simulink model "v2x_cs"  (R2019a)
settings: Solver=ode5  StartTime=0.0  StopTime=inf  FixedStep=1/20  RelTol=1e-3
PreLoadFcn:
  | mbxruntime.callbacks.PreLoadFcn(bdroot);
PostLoadFcn:
  | mbxruntime.callbacks.PostLoadFcn(bdroot);
InitFcn:
  | mbxruntime.callbacks.InitFcn(bdroot);
StartFcn:
  | mbxruntime.callbacks.StartFcn(bdroot);
StopFcn:
  | mbxruntime.callbacks.StopFcn(bdroot);
model workspace (MAT data in the model file):
  mbox_table : struct (value not decoded)
  model_closed = 0
  sim_status = 0
undefined symbols (not defined in the file or in its folder): DiscIntNeverNeededParam, SteeringWheel
libraries: PreScanSimulinkLibrary x10
(part 1 of 5)
CloseFcn:
  | mbxruntime.callbacks.CloseFcn(bdroot);
settings Model: Creator=PRESCAN  LastModifiedBy=DELL
settings DataIOCC: LimitDataPoints=on  SaveFormat=Array  SignalLoggingSaveFormat=ModelDataLogs  ReturnWorkspaceOutputs=off
settings OptimizationCC: ExpressionDepthLimit=2147483647  InitFltsAndDblsToZero=on  LifeSpan=inf
settings DebuggingCC: SaveWithParameterizedLinksMsg=none  UnderspecifiedInitializationDetection=Classic  MergeDetectMultiDrivingBlocksExec=none  SignalResolutionControl=TryResolveAllWithWarning  MultiTaskDSMMsg=warning  MultiTaskCondExecSysMsg=none  FcnCallInpInsideContextMsg=warning  StateNameClashWarn=warning  SFUnexpectedBacktrackingDiag=warning  SFNoUnconditionalDefaultTransitionDiag=warning  SFExecutionAtInitializationDiag=none  ArithmeticOperatorsInVariantConditions=warning
settings HardwareCC: ProdBitPerPointer=32  ProdBitPerSizeT=32  ProdBitPerPtrDiffT=32  ProdLargestAtomicFloat=None  ProdIntDivRoundTo=Undefined  ProdEndianess=Unspecified  ProdWordSize=32  ProdHWDeviceType=32-bit Generic
settings ModelReferenceCC: UpdateModelReferenceTargets=IfOutOfDate  PropagateSignalLabelsOutOfModel=off
settings SFSimCC: SimUseLocalCustomCode=off  SimParseCustomCode=off
settings SFSimCC: SimCustomHeaderCode=|
  | #include "prescan.h"
  | #include "prescan_platform.h"
  | #include "prescan_v2x_data.h"
settings RTWCC: RTWUseLocalCustomCode=off
settings CodeAppCC: StateflowObjectComments=on
settings GRTTargetCC: TargetFcnLib=ansi_tfl_tmw.mat  TargetLangStandard=C89/C90 (ANSI)  GeneratePreprocessorConditionals=Disable all  CombineOutputUpdateFcns=off  GRTInterface=on
settings ConfigComp: CovMetricSettings=dw  CovHtmlReporting=on  CovSaveCumulativeToWorkspaceVar=on  CovSaveSingleToWorkspaceVar=on  CovExternalEMLEnable=off

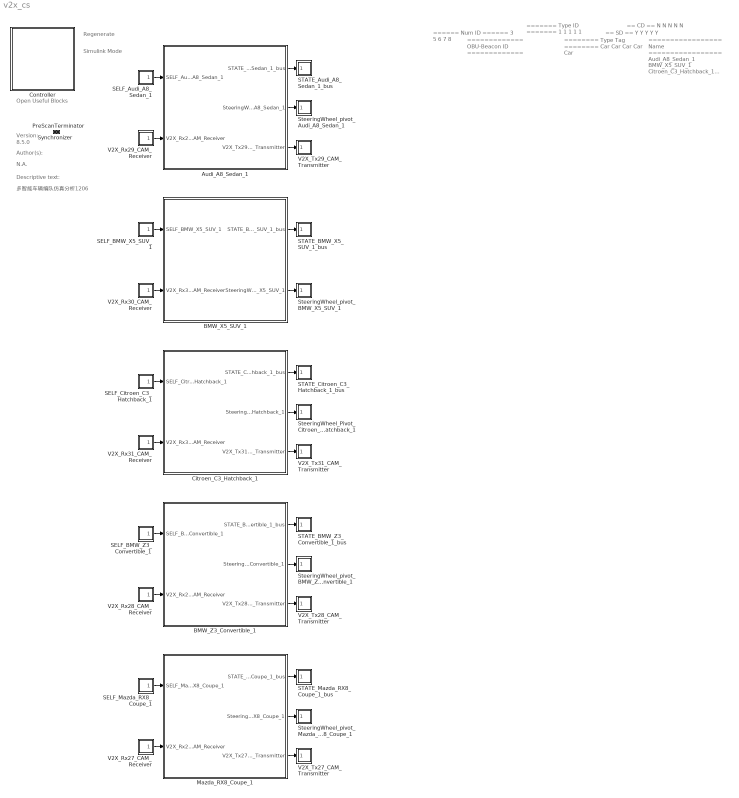
== system v2x_cs ==
  note: Regenerate
  note: Simulink Mode
  note: Open Useful Blocks
  note: 8.5.0
  note: Version:
  note: Author(s):
  note: N.A.
  note: Descriptive text:
  note: 多智能车辆编队仿真分析1206
  note: ======
      | Num ID
      | ======
      | 3
      | 5
      | 6
      | 7
      | 8
  note: =============
      | OBU-Beacon ID
      | =============
  note: =======
      | Type ID
      | =======
      | 1
      | 1
      | 1
      | 1
      | 1
  note: ========
      | Type Tag
      | ========
      | Car
      | Car
      | Car
      | Car
      | Car
  note: ==
      | SD
      | ==
      | Y
      | Y
      | Y
      | Y
      | Y
  note: ==
      | CD
      | ==
      | N
      | N
      | N
      | N
      | N
  note: =================
      | Name
      | =================
      | Audi_A8_Sedan_1
      | BMW_X5_SUV_1
      | Citroen_C3_Hatchback_1
      | BMW_Z3_Convertible_1
      | Mazda_RX8_Coupe_1
  Audi_A8_Sedan_1 : Subsystem  Tag=WorldObjectSubSystem  InitFcn=UniqueId = '22';
      mask init:
      | modelPath = GenericModelHelper.getGenericModelFilePath('ModelDepo','Vehicles\Audi_A8\Audi_A8.pgmb','d771622804618130053427da08a6d484');imagePath = GenericModelHelper.getCompilationPicture(modelPath, 'Audi_A8_HighPoly.png');
      mask Display: image(imread(imagePath));color('white');text(0, 0, ' ID=3\n')
  BMW_X5_SUV_1 : Subsystem  Tag=WorldObjectSubSystem  InitFcn=UniqueId = '23';
      mask init:
      | modelPath = GenericModelHelper.getGenericModelFilePath('ModelDepo','Vehicles\BMW_X5\BMW_X5.pgmb','cea918691563e9ae3e6a88ec95e6726a');imagePath = GenericModelHelper.getCompilationPicture(modelPath, 'BMW_X5_HighPoly.png');
      mask Display: image(imread(imagePath));color('white');text(0, 0, ' ID=5\n')
  BMW_Z3_Convertible_1 : Subsystem  Tag=WorldObjectSubSystem  InitFcn=UniqueId = '25';
      mask init:
      | modelPath = GenericModelHelper.getGenericModelFilePath('ModelDepo','Vehicles\BMW_Z3\BMW_Z3.pgmb','7699e47834166b94c09717861bab4f7a');imagePath = GenericModelHelper.getCompilationPicture(modelPath, 'BMW_Z3_HighPoly.png');
      mask Display: image(imread(imagePath));color('white');text(0, 0, ' ID=7\n')
  Citroen_C3_Hatchback_1 : Subsystem  Tag=WorldObjectSubSystem  InitFcn=UniqueId = '24';
      mask init:
      | modelPath = GenericModelHelper.getGenericModelFilePath('ModelDepo','Vehicles\Citroen_C3\Citroen_C3.pgmb','418afd416d9cb26f62eb87df85de2ab6');imagePath = GenericModelHelper.getCompilationPicture(modelPath, 'Citroen_C3_HighPoly.png');
      mask Display: image(imread(imagePath));color('white');text(0, 0, ' ID=6\n')
  Controller : Subsystem  Description=4395E09780732EACEA18EB3ED2FF7C1B9BEC15E9AB79396025191FD1491BD270  Priority=-1  LoadFcn=load PreScanControllerData  mask(PreScan Simulation Controller){prescanversion='8.5.0', ModelReferencing=off, TimeStep=1/20, ControlMode=0, PreScanExecutionMode=on, ControllerCount=0, ControllerIndex=0, ControllerOptions=''}
      mask prompts: prescanversion "PreScan Version"; ModelReferencing "Use Model Referencing"; TimeStep "Upload Period [s]"; ControlMode "Control Mode"; PreScanExecutionMode "Execution Mode"; ControllerCount "Controller Count"; ControllerIndex "Controller Index"; ControllerOptions "Controller Options"
      mask help:
      | Please do not remove this block from the compilation sheet,
      | as it connects the model to the PreScan environment.
      mask init:
      | model = bdroot(gcb);
      | ExperimentFile = mbxruntime.findExperimentFile(model,true); %relative path
      | 
      | [d1, d2, d3, prescandata] = prescan_Settings();
      | ModelDepo = fullfile(prescandata,'ModelDepo'); 
      | 
      | RTmode = mbxruntime.getRTMode(model);
      | 
      | SimulationMode = get_param(bdroot,'SimulationMode');
      | if strcmp(SimulationMode, 'rapid-accelerator')
      |     SimulationMode = 'external';
      | end
      | TargetName = get_param(bdroot,'SystemTargetFile');
      settings: ModelCloseFcn=assignin('base',['model_closed_' bdroot],true);
      mask Help: eval('openHelp(812)')
      mask Display: image(imread('prescanlogo.ico'))
  Mazda_RX8_Coupe_1 : Subsystem  Tag=WorldObjectSubSystem  InitFcn=UniqueId = '26';
      mask init:
      | modelPath = GenericModelHelper.getGenericModelFilePath('ModelDepo','Vehicles\Mazda_RX8\Mazda_RX8.pgmb','f45c3d42338784d01091d029fcd57bfb');imagePath = GenericModelHelper.getCompilationPicture(modelPath, 'Mazda_RX8_HighPoly.png');
      mask Display: image(imread(imagePath));color('white');text(0, 0, ' ID=8\n')
  PreScanTerminator : Subsystem  Tag=PreScanTerminator  Priority=999  LoadFcn=load PrescanTerminatorData  mask(PreScan Simulation Terminator){TimeStep=1/20}
      mask prompts: TimeStep "Upload Period [s]"
      mask help:
      | Please do not remove this block from the compilation sheet as it
      | connects the model to the PreScan environment.
      mask Help: eval('openHelp(812)')
      mask Display: image(imread('prescanlogo.ico'))
  SELF_Audi_A8_Sedan_1 : Subsystem  Tag=sensor/SelfPort  Priority=3  LoadFcn=load('PreScanSelfSensorData.mat')  mask(PreScan Source Block: SELF){}
      mask help:
      | The SELF port shows (state) information of the actor itself. The outputs are position in the experiment's axis system and the GPS coordinates, and the object's absolute velocity and compass heading.
      |
      | For more information, please click Help.
      settings: OpenFcn=open_system([gcb '/Sensor'],'mask')
      mask Help: eval('openHelp(462)')
      mask Display: image(imread('GPS.png'))
  SELF_BMW_X5_SUV_1 : Subsystem  Tag=sensor/SelfPort  Priority=3  LoadFcn=load('PreScanSelfSensorData.mat')  mask(PreScan Source Block: SELF){}
      mask help:
      | The SELF port shows (state) information of the actor itself. The outputs are position in the experiment's axis system and the GPS coordinates, and the object's absolute velocity and compass heading.
      |
      | For more information, please click Help.
      settings: OpenFcn=open_system([gcb '/Sensor'],'mask')
      mask Help: eval('openHelp(462)')
      mask Display: image(imread('GPS.png'))
  SELF_BMW_Z3_Convertible_1 : Subsystem  Tag=sensor/SelfPort  Priority=3  LoadFcn=load('PreScanSelfSensorData.mat')  mask(PreScan Source Block: SELF){}
      mask help:
      | The SELF port shows (state) information of the actor itself. The outputs are position in the experiment's axis system and the GPS coordinates, and the object's absolute velocity and compass heading.
      |
      | For more information, please click Help.
      settings: OpenFcn=open_system([gcb '/Sensor'],'mask')
      mask Help: eval('openHelp(462)')
      mask Display: image(imread('GPS.png'))
  SELF_Citroen_C3_Hatchback_1 : Subsystem  Tag=sensor/SelfPort  Priority=3  LoadFcn=load('PreScanSelfSensorData.mat')  mask(PreScan Source Block: SELF){}
      mask help:
      | The SELF port shows (state) information of the actor itself. The outputs are position in the experiment's axis system and the GPS coordinates, and the object's absolute velocity and compass heading.
      |
      | For more information, please click Help.
      settings: OpenFcn=open_system([gcb '/Sensor'],'mask')
      mask Help: eval('openHelp(462)')
      mask Display: image(imread('GPS.png'))
  SELF_Mazda_RX8_Coupe_1 : Subsystem  Tag=sensor/SelfPort  Priority=3  LoadFcn=load('PreScanSelfSensorData.mat')  mask(PreScan Source Block: SELF){}
      mask help:
      | The SELF port shows (state) information of the actor itself. The outputs are position in the experiment's axis system and the GPS coordinates, and the object's absolute velocity and compass heading.
      |
      | For more information, please click Help.
      settings: OpenFcn=open_system([gcb '/Sensor'],'mask')
      mask Help: eval('openHelp(462)')
      mask Display: image(imread('GPS.png'))
  STATE_Audi_A8_Sedan_1_bus : Subsystem  Tag=actuator/StatePort  Priority=0  LoadFcn=load('PreScanStateActuatorData.mat')  mask(PreScan Sink Block: State){}
      mask help:
      | The Actor State contains a vector signal of size (9x1), containing the following signals:
      |
      | -  Position    	(x,y,z)             	[m]
      | -  Velocity    	(vx,vy,vz)         	[m/s]
      | -  Angles       	(Roll, Pitch, Yaw)	[rad]
      |
      | The Actor state is defined in the global axis system.
      | The state is superponed on the Initial position defined in the GUI.
      |
      | For more information, please click Help.
      settings: OpenFcn=open_system([gcb '/Actuator'],'mask')
      mask Help: eval('openHelp(222)')
      mask Display: image(imread('State.png'))
  STATE_BMW_X5_SUV_1_bus : Subsystem  Tag=actuator/StatePort  Priority=0  LoadFcn=load('PreScanStateActuatorData.mat')  mask(PreScan Sink Block: State){}
      mask help:
      | The Actor State contains a vector signal of size (9x1), containing the following signals:
      |
      | -  Position    	(x,y,z)             	[m]
      | -  Velocity    	(vx,vy,vz)         	[m/s]
      | -  Angles       	(Roll, Pitch, Yaw)	[rad]
      |
      | The Actor state is defined in the global axis system.
      | The state is superponed on the Initial position defined in the GUI.
      |
      | For more information, please click Help.
      settings: OpenFcn=open_system([gcb '/Actuator'],'mask')
      mask Help: eval('openHelp(222)')
      mask Display: image(imread('State.png'))
  STATE_BMW_Z3_Convertible_1_bus : Subsystem  Tag=actuator/StatePort  Priority=0  LoadFcn=load('PreScanStateActuatorData.mat')  mask(PreScan Sink Block: State){}
      mask help:
      | The Actor State contains a vector signal of size (9x1), containing the following signals:
      |
      | -  Position    	(x,y,z)             	[m]
      | -  Velocity    	(vx,vy,vz)         	[m/s]
      | -  Angles       	(Roll, Pitch, Yaw)	[rad]
      |
      | The Actor state is defined in the global axis system.
      | The state is superponed on the Initial position defined in the GUI.
      |
      | For more information, please click Help.
      settings: OpenFcn=open_system([gcb '/Actuator'],'mask')
      mask Help: eval('openHelp(222)')
      mask Display: image(imread('State.png'))
  STATE_Citroen_C3_Hatchback_1_bus : Subsystem  Tag=actuator/StatePort  Priority=0  LoadFcn=load('PreScanStateActuatorData.mat')  mask(PreScan Sink Block: State){}
      mask help:
      | The Actor State contains a vector signal of size (9x1), containing the following signals:
      |
      | -  Position    	(x,y,z)             	[m]
      | -  Velocity    	(vx,vy,vz)         	[m/s]
      | -  Angles       	(Roll, Pitch, Yaw)	[rad]
      |
      | The Actor state is defined in the global axis system.
      | The state is superponed on the Initial position defined in the GUI.
      |
      | For more information, please click Help.
      settings: OpenFcn=open_system([gcb '/Actuator'],'mask')
      mask Help: eval('openHelp(222)')
      mask Display: image(imread('State.png'))
  STATE_Mazda_RX8_Coupe_1_bus : Subsystem  Tag=actuator/StatePort  Priority=0  LoadFcn=load('PreScanStateActuatorData.mat')  mask(PreScan Sink Block: State){}
      mask help:
      | The Actor State contains a vector signal of size (9x1), containing the following signals:
      |
      | -  Position    	(x,y,z)             	[m]
      | -  Velocity    	(vx,vy,vz)         	[m/s]
      | -  Angles       	(Roll, Pitch, Yaw)	[rad]
      |
      | The Actor state is defined in the global axis system.
      | The state is superponed on the Initial position defined in the GUI.
      |
      | For more information, please click Help.
      settings: OpenFcn=open_system([gcb '/Actuator'],'mask')
      mask Help: eval('openHelp(222)')
      mask Display: image(imread('State.png'))
  SteeringWheel_Pivot_Citroen_C3_Hatchback_1 : Subsystem  Tag=Actuator  Priority=0  LoadFcn=load('PrescanPoseData');load('PrescanXYZData');load('PreScanRPYData')
      mask help:
      | The VisuJoint block provides a way to adapt the location and orientation of a part of an object.
      |
      | For more information, please click Help.
      settings: OpenFcn=open_system([gcb '/Actuator'],'mask')
      mask Display: image(imread('Joint.png'))
  SteeringWheel_pivot_Audi_A8_Sedan_1 : Subsystem  Tag=Actuator  Priority=0  LoadFcn=load('PrescanPoseData');load('PrescanXYZData');load('PreScanRPYData')
      mask help:
      | The VisuJoint block provides a way to adapt the location and orientation of a part of an object.
      |
      | For more information, please click Help.
      settings: OpenFcn=open_system([gcb '/Actuator'],'mask')
      mask Display: image(imread('Joint.png'))
  SteeringWheel_pivot_BMW_X5_SUV_1 : Subsystem  Tag=Actuator  Priority=0  LoadFcn=load('PrescanPoseData');load('PrescanXYZData');load('PreScanRPYData')
      mask help:
      | The VisuJoint block provides a way to adapt the location and orientation of a part of an object.
      |
      | For more information, please click Help.
      settings: OpenFcn=open_system([gcb '/Actuator'],'mask')
      mask Display: image(imread('Joint.png'))
  SteeringWheel_pivot_BMW_Z3_Convertible_1 : Subsystem  Tag=Actuator  Priority=0  LoadFcn=load('PrescanPoseData');load('PrescanXYZData');load('PreScanRPYData')
      mask help:
      | The VisuJoint block provides a way to adapt the location and orientation of a part of an object.
      |
      | For more information, please click Help.
      settings: OpenFcn=open_system([gcb '/Actuator'],'mask')
      mask Display: image(imread('Joint.png'))
  SteeringWheel_pivot_Mazda_RX8_Coupe_1 : Subsystem  Tag=Actuator  Priority=0  LoadFcn=load('PrescanPoseData');load('PrescanXYZData');load('PreScanRPYData')
      mask help:
      | The VisuJoint block provides a way to adapt the location and orientation of a part of an object.
      |
      | For more information, please click Help.
      settings: OpenFcn=open_system([gcb '/Actuator'],'mask')
      mask Display: image(imread('Joint.png'))
  Synchronizer : Subsystem  Tag=PreScanSynchronizer  Priority=1  LoadFcn=load PrescanSynchronizeData  mask(PreScan Simulation Core Block){TimeStep=1/20}
      mask prompts: TimeStep "Timestep [s]"
      mask help:
      | Please do not remove this block from the PreScan compilation sheet,
      | as it contains essential configuration parameters for a PreScan simulation.
      settings: DeleteFcn=PreScanBlockDeleteFcn;
      mask Display: image(imread('prescanlogo.ico'))
  V2X_Rx27_CAM_Receiver : Subsystem  Tag=sensor/plugin/sfun_V2X_CAM_Receiver  Priority=3  mask(V2X CAM Receiver Block){}
      mask help: V2X Block receiving a CAM message
      settings: OpenFcn=open_system([gcb '/Sensor'],'mask')
      mask Help: eval('openHelp()')
      mask Display: image(imread('V2XR_grayscale.png'))
  V2X_Rx28_CAM_Receiver : Subsystem  Tag=sensor/plugin/sfun_V2X_CAM_Receiver  Priority=3  mask(V2X CAM Receiver Block){}
      mask help: V2X Block receiving a CAM message
      settings: OpenFcn=open_system([gcb '/Sensor'],'mask')
      mask Help: eval('openHelp()')
      mask Display: image(imread('V2XR_grayscale.png'))
  V2X_Rx29_CAM_Receiver : Subsystem  Tag=sensor/plugin/sfun_V2X_CAM_Receiver  Priority=3  mask(V2X CAM Receiver Block){}
      mask help: V2X Block receiving a CAM message
      settings: OpenFcn=open_system([gcb '/Sensor'],'mask')
      mask Help: eval('openHelp()')
      mask Display: image(imread('V2XR_grayscale.png'))
  V2X_Rx30_CAM_Receiver : Subsystem  Tag=sensor/plugin/sfun_V2X_CAM_Receiver  Priority=3  mask(V2X CAM Receiver Block){}
      mask help: V2X Block receiving a CAM message
      settings: OpenFcn=open_system([gcb '/Sensor'],'mask')
      mask Help: eval('openHelp()')
      mask Display: image(imread('V2XR_grayscale.png'))
  V2X_Rx31_CAM_Receiver : Subsystem  Tag=sensor/plugin/sfun_V2X_CAM_Receiver  Priority=3  mask(V2X CAM Receiver Block){}
      mask help: V2X Block receiving a CAM message
      settings: OpenFcn=open_system([gcb '/Sensor'],'mask')
      mask Help: eval('openHelp()')
      mask Display: image(imread('V2XR_grayscale.png'))
  V2X_Tx27_CAM_Transmitter : Subsystem  Tag=actuator/plugin/sfun_V2X_CAM_Transmitter  Priority=0  mask(V2X CAM Transmitter Block){}
      mask help: V2X Block transmitting a CAM message
      settings: OpenFcn=open_system([gcb '/Actuator'],'mask')
      mask Help: eval('openHelp()')
      mask Display: image(imread('V2XT_grayscale.png'))
  V2X_Tx28_CAM_Transmitter : Subsystem  Tag=actuator/plugin/sfun_V2X_CAM_Transmitter  Priority=0  mask(V2X CAM Transmitter Block){}
      mask help: V2X Block transmitting a CAM message
      settings: OpenFcn=open_system([gcb '/Actuator'],'mask')
      mask Help: eval('openHelp()')
      mask Display: image(imread('V2XT_grayscale.png'))
  V2X_Tx29_CAM_Transmitter : Subsystem  Tag=actuator/plugin/sfun_V2X_CAM_Transmitter  Priority=0  mask(V2X CAM Transmitter Block){}
      mask help: V2X Block transmitting a CAM message
      settings: OpenFcn=open_system([gcb '/Actuator'],'mask')
      mask Help: eval('openHelp()')
      mask Display: image(imread('V2XT_grayscale.png'))
  V2X_Tx31_CAM_Transmitter : Subsystem  Tag=actuator/plugin/sfun_V2X_CAM_Transmitter  Priority=0  mask(V2X CAM Transmitter Block){}
      mask help: V2X Block transmitting a CAM message
      settings: OpenFcn=open_system([gcb '/Actuator'],'mask')
      mask Help: eval('openHelp()')
      mask Display: image(imread('V2XT_grayscale.png'))
  wires:
  Audi_A8_Sedan_1/1(STATE_Audi_A8_Sedan_1_bus) -> STATE_Audi_A8_Sedan_1_bus/1(STATE_Audi_A8_Sedan_1_bus)
  SELF_Audi_A8_Sedan_1/1(SELF_Audi_A8_Sedan_1) -> Audi_A8_Sedan_1/1(SELF_Audi_A8_Sedan_1)
  Audi_A8_Sedan_1/2(SteeringWheel_pivot_Audi_A8_Sedan_1) -> SteeringWheel_pivot_Audi_A8_Sedan_1/1(SteeringWheel_pivot_Audi_A8_Sedan_1)
  Audi_A8_Sedan_1/3(V2X_Tx29_CAM_Transmitter) -> V2X_Tx29_CAM_Transmitter/1(V2X_Tx29_CAM_Transmitter)
  V2X_Rx29_CAM_Receiver/1(V2X_Rx29_CAM_Receiver) -> Audi_A8_Sedan_1/2(V2X_Rx29_CAM_Receiver)
  BMW_X5_SUV_1/1(STATE_BMW_X5_SUV_1_bus) -> STATE_BMW_X5_SUV_1_bus/1(STATE_BMW_X5_SUV_1_bus)
  SELF_BMW_X5_SUV_1/1(SELF_BMW_X5_SUV_1) -> BMW_X5_SUV_1/1(SELF_BMW_X5_SUV_1)
  BMW_X5_SUV_1/2(SteeringWheel_pivot_BMW_X5_SUV_1) -> SteeringWheel_pivot_BMW_X5_SUV_1/1(SteeringWheel_pivot_BMW_X5_SUV_1)
  V2X_Rx30_CAM_Receiver/1(V2X_Rx30_CAM_Receiver) -> BMW_X5_SUV_1/2(V2X_Rx30_CAM_Receiver)
  Citroen_C3_Hatchback_1/1(STATE_Citroen_C3_Hatchback_1_bus) -> STATE_Citroen_C3_Hatchback_1_bus/1(STATE_Citroen_C3_Hatchback_1_bus)
  SELF_Citroen_C3_Hatchback_1/1(SELF_Citroen_C3_Hatchback_1) -> Citroen_C3_Hatchback_1/1(SELF_Citroen_C3_Hatchback_1)
  Citroen_C3_Hatchback_1/2(SteeringWheel_Pivot_Citroen_C3_Hatchback_1) -> SteeringWheel_Pivot_Citroen_C3_Hatchback_1/1(SteeringWheel_Pivot_Citroen_C3_Hatchback_1)
  Citroen_C3_Hatchback_1/3(V2X_Tx31_CAM_Transmitter) -> V2X_Tx31_CAM_Transmitter/1(V2X_Tx31_CAM_Transmitter)
  V2X_Rx31_CAM_Receiver/1(V2X_Rx31_CAM_Receiver) -> Citroen_C3_Hatchback_1/2(V2X_Rx31_CAM_Receiver)
  BMW_Z3_Convertible_1/1(STATE_BMW_Z3_Convertible_1_bus) -> STATE_BMW_Z3_Convertible_1_bus/1(STATE_BMW_Z3_Convertible_1_bus)
  SELF_BMW_Z3_Convertible_1/1(SELF_BMW_Z3_Convertible_1) -> BMW_Z3_Convertible_1/1(SELF_BMW_Z3_Convertible_1)
  BMW_Z3_Convertible_1/2(SteeringWheel_pivot_BMW_Z3_Convertible_1) -> SteeringWheel_pivot_BMW_Z3_Convertible_1/1(SteeringWheel_pivot_BMW_Z3_Convertible_1)
  BMW_Z3_Convertible_1/3(V2X_Tx28_CAM_Transmitter) -> V2X_Tx28_CAM_Transmitter/1(V2X_Tx28_CAM_Transmitter)
  V2X_Rx28_CAM_Receiver/1(V2X_Rx28_CAM_Receiver) -> BMW_Z3_Convertible_1/2(V2X_Rx28_CAM_Receiver)
  Mazda_RX8_Coupe_1/1(STATE_Mazda_RX8_Coupe_1_bus) -> STATE_Mazda_RX8_Coupe_1_bus/1(STATE_Mazda_RX8_Coupe_1_bus)
  SELF_Mazda_RX8_Coupe_1/1(SELF_Mazda_RX8_Coupe_1) -> Mazda_RX8_Coupe_1/1(SELF_Mazda_RX8_Coupe_1)
  Mazda_RX8_Coupe_1/2(SteeringWheel_pivot_Mazda_RX8_Coupe_1) -> SteeringWheel_pivot_Mazda_RX8_Coupe_1/1(SteeringWheel_pivot_Mazda_RX8_Coupe_1)
  Mazda_RX8_Coupe_1/3(V2X_Tx27_CAM_Transmitter) -> V2X_Tx27_CAM_Transmitter/1(V2X_Tx27_CAM_Transmitter)
  V2X_Rx27_CAM_Receiver/1(V2X_Rx27_CAM_Receiver) -> Mazda_RX8_Coupe_1/2(V2X_Rx27_CAM_Receiver)

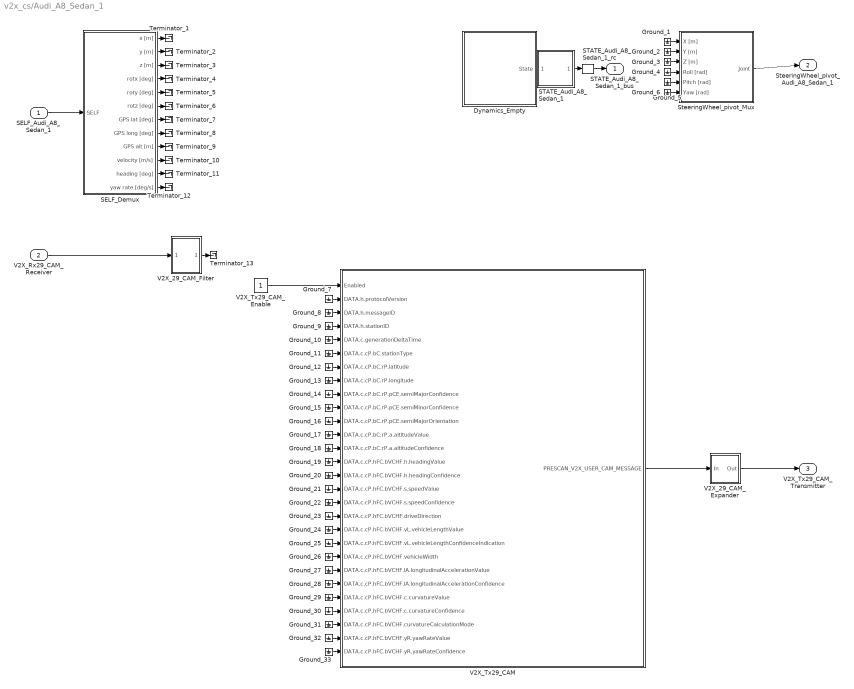
== system v2x_cs/Audi_A8_Sedan_1 ==
  SELF_Audi_A8_Sedan_1 : Inport  Tag=inport/SelfPort  OutDataTypeStr=Bus: PRESCAN_SELFSENSORDATA  PortDimensions=1  SampleTime=1/20  BusOutputAsStruct=on
  V2X_Rx29_CAM_Receiver : Inport  Tag=inport/plugin/sfun_V2X_CAM_Receiver  Port=2  BusOutputAsStruct=on
  Dynamics_Empty : Subsystem  Tag=Dynamics_Empty
      mask Help: eval('openHelp(202)')
      mask Display: port_label('output', 1, 'State');text(0,0,' Empty\n')
  Ground_{1..33} (33 alike) : Ground
  SELF_Demux : Subsystem  Tag=demux/SelfPort  mask(PreScan Demux Block:){}
      mask help:
      | The SELF port shows (state) information of the actor itself. The outputs are position in the experiment's axis system and the GPS coordinates, and the object's absolute velocity and compass heading.
      |
      | For more information, please click Help.
      settings: DeleteFcn=PreScanBlockDeleteFcn;
      mask Help: eval('openHelp(462)')
      mask Display:
      | port_label('output',1,'x [m]')
      | port_label('output',2,'y [m]')
      | port_label('output',3,'z [m]','texmode','on')
      | port_label('output',4,'Rotx [deg]','texmode','on')
      | port_label('output',5,'Roty [deg]','texmode','on')
      | port_label('output',6,'Rotz [deg]','texmode','on')
      | port_label('output',7,'GPS lat [deg]','texmode','on')
      | port_label('output',8,'GPS long [deg]','texmode','on')
      | port_label('output',9,'GPS alt [m]','texmode','on')
      | port_label('output',10,'Velocity [m/s]')
      | port_label('output',11,'Heading [deg]')
      | port_label('output',12,'Yaw rate [deg/s]')
  STATE_Audi_A8_Sedan_1 : Subsystem  Tag=mux/StatePort  Priority=0  LoadFcn=load PrescanStateActuatorData  mask(PreScan Sink Block: State){x0=21.3511, y0=5.4609, z0=0.55, Roll0=0, Pitch0=0, Yaw0=0, TimeStep=1/20}
      mask prompts: x0 "Ini x-position VEHICLE wrt GLOBAL axis system [m]"; y0 "Ini y-position VEHICLE wrt GLOBAL axis system [m]"; z0 "Ini z-position VEHICLE wrt GLOBAL axis system [m]"; Roll0 "Ini roll-angle BODY wrt VEHICLE axis system [deg]"; Pitch0 "Ini pitch-angle BODY wrt VEHICLE axis system [deg]"; Yaw0 "Ini yaw-angle VEHICLE wrt GLOBAL axis system [deg]"; TimeStep "Auto-Assigned: Upload Period [s]"
      mask help:
      | The Actor State contains a vector signal of size (9x1), containing the following signals:
      |
      | -  Position                  (x,y,z)                                     [m]
      | -  Velocity                  (vx,vy,vz)                               [m/s]
      | -  Angles                    (Roll, Pitch, Yaw)                   [rad]
      |
      | The Actor state is defined in the global axis system.
      | The state is superponed on the Initial position defined in the GUI.
      |
      | For more information, please click Help.
      settings: DeleteFcn=PreScanBlockDeleteFcn;
      mask Help: eval('openHelp(222)')
      mask Display: image(imread('State.png'))
  STATE_Audi_A8_Sedan_1_rc : RateTransition  Tag=mux_rc/StatePort  OutPortSampleTimeOpt=Inherit
  SteeringWheel_pivot_Mux : Subsystem  Tag=mux/Joint  mask(PreScan Mux Block){DisplayName=SteeringWheel}
      mask prompts: DisplayName "Display Name"
      mask help:
      | This block simulates a generic joint used for generic models. This joint can be enabled/disabled from the GUI.
      |
      | For more information, please click Help.
      settings: DeleteFcn=PreScanBlockDeleteFcn;
      mask Help: eval('openHelp(254)')
  Terminator_{1..13} (13 alike) : Terminator
  V2X_29_CAM_Expander : Subsystem  LoadFcn=addpath .\V2XPlugin; V2Xbusses;
  V2X_29_CAM_Filter : Subsystem
      mask Display: disp('[3]');
  V2X_Tx29_CAM : Subsystem
  V2X_Tx29_CAM_Enable : Constant  OutDataTypeStr=Inherit: Inherit via back propagation
  STATE_Audi_A8_Sedan_1_bus : Outport  Tag=outport/StatePort  OutDataTypeStr=Bus: PRESCAN_STATEACTUATORDATA  PortDimensions=1  SampleTime=1/20
  SteeringWheel_pivot_Audi_A8_Sedan_1 : Outport  Tag=outport/JointActuator  Port=2  OutDataTypeStr=Bus: PRESCAN_POSE_DATA  SampleTime=1/20
  V2X_Tx29_CAM_Transmitter : Outport  Tag=outport/plugin/sfun_V2X_CAM_Transmitter  Port=3
  wires:
  STATE_Audi_A8_Sedan_1_rc/1 -> STATE_Audi_A8_Sedan_1_bus/1
  STATE_Audi_A8_Sedan_1/1(StateBus) -> STATE_Audi_A8_Sedan_1_rc/1
  SELF_Audi_A8_Sedan_1/1 -> SELF_Demux/1(SELF)
  SteeringWheel_pivot_Mux/1(Joint) -> SteeringWheel_pivot_Audi_A8_Sedan_1/1
  Dynamics_Empty/1(State) -> STATE_Audi_A8_Sedan_1/1(State)
  V2X_Tx29_CAM_Enable/1 -> V2X_Tx29_CAM/1(Enabled)
  V2X_Tx29_CAM/1(PRESCAN_V2X_USER_CAM_MESSAGE) -> V2X_29_CAM_Expander/1(In)
  V2X_29_CAM_Expander/1(Out) -> V2X_Tx29_CAM_Transmitter/1
  V2X_Rx29_CAM_Receiver/1 -> V2X_29_CAM_Filter/1(Filter_In)
  SELF_Demux/1(x [m]) -> Terminator_1/1
  SELF_Demux/2(y [m]) -> Terminator_2/1
  SELF_Demux/3(z [m]) -> Terminator_3/1
  SELF_Demux/4(rotx [deg]) -> Terminator_4/1
  SELF_Demux/5(roty [deg]) -> Terminator_5/1
  SELF_Demux/6(rotz [deg]) -> Terminator_6/1
  SELF_Demux/7(GPS lat [deg]) -> Terminator_7/1
  SELF_Demux/8(GPS long [deg]) -> Terminator_8/1
  SELF_Demux/9(GPS alt [m]) -> Terminator_9/1
  SELF_Demux/10(velocity [m/s]) -> Terminator_10/1
  SELF_Demux/11(heading [deg]) -> Terminator_11/1
  SELF_Demux/12(yaw rate [deg/s]) -> Terminator_12/1
  Ground_1/1 -> SteeringWheel_pivot_Mux/1(X [m])
  Ground_2/1 -> SteeringWheel_pivot_Mux/2(Y [m])
  Ground_3/1 -> SteeringWheel_pivot_Mux/3(Z [m])
  Ground_4/1 -> SteeringWheel_pivot_Mux/4(Roll [rad])
  Ground_5/1 -> SteeringWheel_pivot_Mux/5(Pitch [rad])
  Ground_6/1 -> SteeringWheel_pivot_Mux/6(Yaw [rad])
  V2X_29_CAM_Filter/1(Filter_Out) -> Terminator_13/1
  Ground_7/1 -> V2X_Tx29_CAM/2(DATA.h.protocolVersion)
  Ground_8/1 -> V2X_Tx29_CAM/3(DATA.h.messageID)
  Ground_9/1 -> V2X_Tx29_CAM/4(DATA.h.stationID)
  Ground_10/1 -> V2X_Tx29_CAM/5(DATA.c.generationDeltaTime)
  Ground_11/1 -> V2X_Tx29_CAM/6(DATA.c.cP.bC.stationType)
  Ground_12/1 -> V2X_Tx29_CAM/7(DATA.c.cP.bC.rP.latitude)
  Ground_13/1 -> V2X_Tx29_CAM/8(DATA.c.cP.bC.rP.longitude)
  Ground_14/1 -> V2X_Tx29_CAM/9(DATA.c.cP.bC.rP.pCE.semiMajorConfidence)
  Ground_15/1 -> V2X_Tx29_CAM/10(DATA.c.cP.bC.rP.pCE.semiMinorConfidence)
  Ground_16/1 -> V2X_Tx29_CAM/11(DATA.c.cP.bC.rP.pCE.semiMajorOrientation)
  Ground_17/1 -> V2X_Tx29_CAM/12(DATA.c.cP.bC.rP.a.altitudeValue)
  Ground_18/1 -> V2X_Tx29_CAM/13(DATA.c.cP.bC.rP.a.altitudeConfidence)
  Ground_19/1 -> V2X_Tx29_CAM/14(DATA.c.cP.hFC.bVCHF.h.headingValue)
  Ground_20/1 -> V2X_Tx29_CAM/15(DATA.c.cP.hFC.bVCHF.h.headingConfidence)
  Ground_21/1 -> V2X_Tx29_CAM/16(DATA.c.cP.hFC.bVCHF.s.speedValue)
  Ground_22/1 -> V2X_Tx29_CAM/17(DATA.c.cP.hFC.bVCHF.s.speedConfidence)
  Ground_23/1 -> V2X_Tx29_CAM/18(DATA.c.cP.hFC.bVCHF.driveDirection)
  Ground_24/1 -> V2X_Tx29_CAM/19(DATA.c.cP.hFC.bVCHF.vL.vehicleLengthValue)
  Ground_25/1 -> V2X_Tx29_CAM/20(DATA.c.cP.hFC.bVCHF.vL.vehicleLengthConfidenceIndication)
  Ground_26/1 -> V2X_Tx29_CAM/21(DATA.c.cP.hFC.bVCHF.vehicleWidth)
  Ground_27/1 -> V2X_Tx29_CAM/22(DATA.c.cP.hFC.bVCHF.lA.longitudinalAccelerationValue)
  Ground_28/1 -> V2X_Tx29_CAM/23(DATA.c.cP.hFC.bVCHF.lA.longitudinalAccelerationConfidence)
  Ground_29/1 -> V2X_Tx29_CAM/24(DATA.c.cP.hFC.bVCHF.c.curvatureValue)
  Ground_30/1 -> V2X_Tx29_CAM/25(DATA.c.cP.hFC.bVCHF.c.curvatureConfidence)
  Ground_31/1 -> V2X_Tx29_CAM/26(DATA.c.cP.hFC.bVCHF.curvatureCalculationMode)
  Ground_32/1 -> V2X_Tx29_CAM/27(DATA.c.cP.hFC.bVCHF.yR.yawRateValue)
  Ground_33/1 -> V2X_Tx29_CAM/28(DATA.c.cP.hFC.bVCHF.yR.yawRateConfidence)

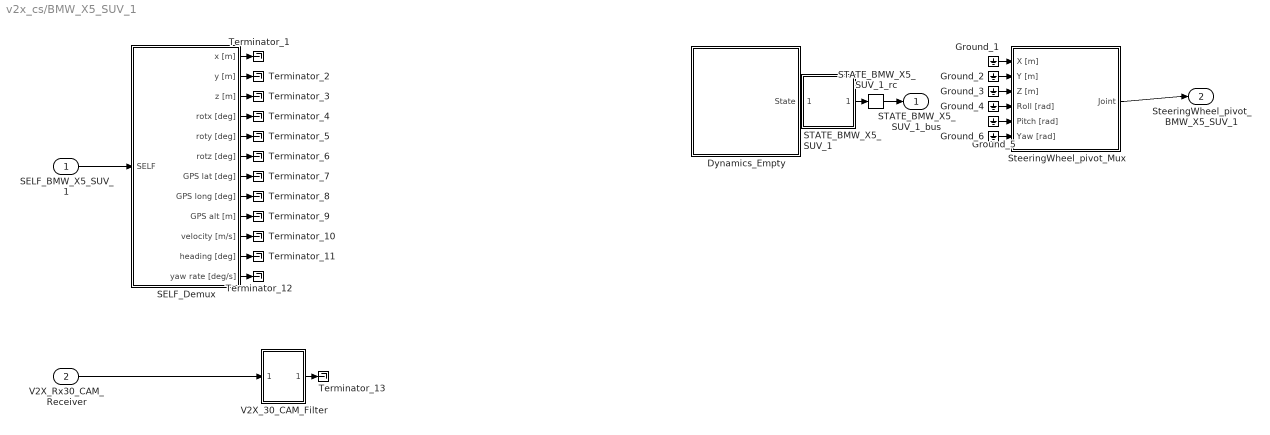
== system v2x_cs/BMW_X5_SUV_1 ==
  SELF_BMW_X5_SUV_1 : Inport  Tag=inport/SelfPort  OutDataTypeStr=Bus: PRESCAN_SELFSENSORDATA  PortDimensions=1  SampleTime=1/20  BusOutputAsStruct=on
  V2X_Rx30_CAM_Receiver : Inport  Tag=inport/plugin/sfun_V2X_CAM_Receiver  Port=2  BusOutputAsStruct=on
  Dynamics_Empty : Subsystem  Tag=Dynamics_Empty
      mask Help: eval('openHelp(202)')
      mask Display: port_label('output', 1, 'State');text(0,0,' Empty\n')
  Ground_{1..6} (6 alike) : Ground
  SELF_Demux : Subsystem  Tag=demux/SelfPort  mask(PreScan Demux Block:){}
      mask help:
      | The SELF port shows (state) information of the actor itself. The outputs are position in the experiment's axis system and the GPS coordinates, and the object's absolute velocity and compass heading.
      |
      | For more information, please click Help.
      settings: DeleteFcn=PreScanBlockDeleteFcn;
      mask Help: eval('openHelp(462)')
      mask Display:
      | port_label('output',1,'x [m]')
      | port_label('output',2,'y [m]')
      | port_label('output',3,'z [m]','texmode','on')
      | port_label('output',4,'Rotx [deg]','texmode','on')
      | port_label('output',5,'Roty [deg]','texmode','on')
      | port_label('output',6,'Rotz [deg]','texmode','on')
      | port_label('output',7,'GPS lat [deg]','texmode','on')
      | port_label('output',8,'GPS long [deg]','texmode','on')
      | port_label('output',9,'GPS alt [m]','texmode','on')
      | port_label('output',10,'Velocity [m/s]')
      | port_label('output',11,'Heading [deg]')
      | port_label('output',12,'Yaw rate [deg/s]')
  STATE_BMW_X5_SUV_1 : Subsystem  Tag=mux/StatePort  Priority=0  LoadFcn=load PrescanStateActuatorData  mask(PreScan Sink Block: State){x0=5.7069, y0=-1.6042, z0=0.69, Roll0=0, Pitch0=0, Yaw0=0, TimeStep=1/20}
      mask prompts: x0 "Ini x-position VEHICLE wrt GLOBAL axis system [m]"; y0 "Ini y-position VEHICLE wrt GLOBAL axis system [m]"; z0 "Ini z-position VEHICLE wrt GLOBAL axis system [m]"; Roll0 "Ini roll-angle BODY wrt VEHICLE axis system [deg]"; Pitch0 "Ini pitch-angle BODY wrt VEHICLE axis system [deg]"; Yaw0 "Ini yaw-angle VEHICLE wrt GLOBAL axis system [deg]"; TimeStep "Auto-Assigned: Upload Period [s]"
      mask help:
      | The Actor State contains a vector signal of size (9x1), containing the following signals:
      |
      | -  Position                  (x,y,z)                                     [m]
      | -  Velocity                  (vx,vy,vz)                               [m/s]
      | -  Angles                    (Roll, Pitch, Yaw)                   [rad]
      |
      | The Actor state is defined in the global axis system.
      | The state is superponed on the Initial position defined in the GUI.
      |
      | For more information, please click Help.
      settings: DeleteFcn=PreScanBlockDeleteFcn;
      mask Help: eval('openHelp(222)')
      mask Display: image(imread('State.png'))
  STATE_BMW_X5_SUV_1_rc : RateTransition  Tag=mux_rc/StatePort  OutPortSampleTimeOpt=Inherit
  SteeringWheel_pivot_Mux : Subsystem  Tag=mux/Joint  mask(PreScan Mux Block){DisplayName=SteeringWheel}
      mask prompts: DisplayName "Display Name"
      mask help:
      | This block simulates a generic joint used for generic models. This joint can be enabled/disabled from the GUI.
      |
      | For more information, please click Help.
      settings: DeleteFcn=PreScanBlockDeleteFcn;
      mask Help: eval('openHelp(254)')
  Terminator_{1..13} (13 alike) : Terminator
  V2X_30_CAM_Filter : Subsystem
      mask Display: disp('[4]');
  STATE_BMW_X5_SUV_1_bus : Outport  Tag=outport/StatePort  OutDataTypeStr=Bus: PRESCAN_STATEACTUATORDATA  PortDimensions=1  SampleTime=1/20
  SteeringWheel_pivot_BMW_X5_SUV_1 : Outport  Tag=outport/JointActuator  Port=2  OutDataTypeStr=Bus: PRESCAN_POSE_DATA  SampleTime=1/20
  wires:
  STATE_BMW_X5_SUV_1_rc/1 -> STATE_BMW_X5_SUV_1_bus/1
  STATE_BMW_X5_SUV_1/1(StateBus) -> STATE_BMW_X5_SUV_1_rc/1
  SELF_BMW_X5_SUV_1/1 -> SELF_Demux/1(SELF)
  SteeringWheel_pivot_Mux/1(Joint) -> SteeringWheel_pivot_BMW_X5_SUV_1/1
  Dynamics_Empty/1(State) -> STATE_BMW_X5_SUV_1/1(State)
  V2X_Rx30_CAM_Receiver/1 -> V2X_30_CAM_Filter/1(Filter_In)
  SELF_Demux/1(x [m]) -> Terminator_1/1
  SELF_Demux/2(y [m]) -> Terminator_2/1
  SELF_Demux/3(z [m]) -> Terminator_3/1
  SELF_Demux/4(rotx [deg]) -> Terminator_4/1
  SELF_Demux/5(roty [deg]) -> Terminator_5/1
  SELF_Demux/6(rotz [deg]) -> Terminator_6/1
  SELF_Demux/7(GPS lat [deg]) -> Terminator_7/1
  SELF_Demux/8(GPS long [deg]) -> Terminator_8/1
  SELF_Demux/9(GPS alt [m]) -> Terminator_9/1
  SELF_Demux/10(velocity [m/s]) -> Terminator_10/1
  SELF_Demux/11(heading [deg]) -> Terminator_11/1
  SELF_Demux/12(yaw rate [deg/s]) -> Terminator_12/1
  Ground_1/1 -> SteeringWheel_pivot_Mux/1(X [m])
  Ground_2/1 -> SteeringWheel_pivot_Mux/2(Y [m])
  Ground_3/1 -> SteeringWheel_pivot_Mux/3(Z [m])
  Ground_4/1 -> SteeringWheel_pivot_Mux/4(Roll [rad])
  Ground_5/1 -> SteeringWheel_pivot_Mux/5(Pitch [rad])
  Ground_6/1 -> SteeringWheel_pivot_Mux/6(Yaw [rad])
  V2X_30_CAM_Filter/1(Filter_Out) -> Terminator_13/1

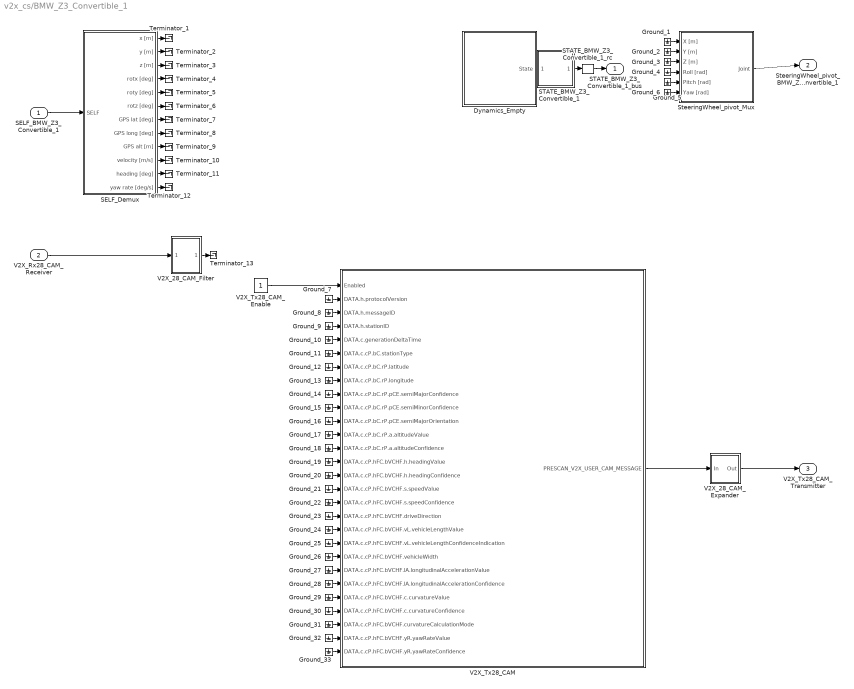
== system v2x_cs/BMW_Z3_Convertible_1 ==
  SELF_BMW_Z3_Convertible_1 : Inport  Tag=inport/SelfPort  OutDataTypeStr=Bus: PRESCAN_SELFSENSORDATA  PortDimensions=1  SampleTime=1/20  BusOutputAsStruct=on
  V2X_Rx28_CAM_Receiver : Inport  Tag=inport/plugin/sfun_V2X_CAM_Receiver  Port=2  BusOutputAsStruct=on
  Dynamics_Empty : Subsystem  Tag=Dynamics_Empty
      mask Help: eval('openHelp(202)')
      mask Display: port_label('output', 1, 'State');text(0,0,' Empty\n')
  Ground_{1..33} (33 alike) : Ground
  SELF_Demux : Subsystem  Tag=demux/SelfPort  mask(PreScan Demux Block:){}
      mask help:
      | The SELF port shows (state) information of the actor itself. The outputs are position in the experiment's axis system and the GPS coordinates, and the object's absolute velocity and compass heading.
      |
      | For more information, please click Help.
      settings: DeleteFcn=PreScanBlockDeleteFcn;
      mask Help: eval('openHelp(462)')
      mask Display:
      | port_label('output',1,'x [m]')
      | port_label('output',2,'y [m]')
      | port_label('output',3,'z [m]','texmode','on')
      | port_label('output',4,'Rotx [deg]','texmode','on')
      | port_label('output',5,'Roty [deg]','texmode','on')
      | port_label('output',6,'Rotz [deg]','texmode','on')
      | port_label('output',7,'GPS lat [deg]','texmode','on')
      | port_label('output',8,'GPS long [deg]','texmode','on')
      | port_label('output',9,'GPS alt [m]','texmode','on')
      | port_label('output',10,'Velocity [m/s]')
      | port_label('output',11,'Heading [deg]')
      | port_label('output',12,'Yaw rate [deg/s]')
  STATE_BMW_Z3_Convertible_1 : Subsystem  Tag=mux/StatePort  Priority=0  LoadFcn=load PrescanStateActuatorData  mask(PreScan Sink Block: State){x0=44.8173, y0=2.1807, z0=0.4784, Roll0=0, Pitch0=0, Yaw0=0, TimeStep=1/20}
      mask prompts: x0 "Ini x-position VEHICLE wrt GLOBAL axis system [m]"; y0 "Ini y-position VEHICLE wrt GLOBAL axis system [m]"; z0 "Ini z-position VEHICLE wrt GLOBAL axis system [m]"; Roll0 "Ini roll-angle BODY wrt VEHICLE axis system [deg]"; Pitch0 "Ini pitch-angle BODY wrt VEHICLE axis system [deg]"; Yaw0 "Ini yaw-angle VEHICLE wrt GLOBAL axis system [deg]"; TimeStep "Auto-Assigned: Upload Period [s]"
      mask help:
      | The Actor State contains a vector signal of size (9x1), containing the following signals:
      |
      | -  Position                  (x,y,z)                                     [m]
      | -  Velocity                  (vx,vy,vz)                               [m/s]
      | -  Angles                    (Roll, Pitch, Yaw)                   [rad]
      |
      | The Actor state is defined in the global axis system.
      | The state is superponed on the Initial position defined in the GUI.
      |
      | For more information, please click Help.
      settings: DeleteFcn=PreScanBlockDeleteFcn;
      mask Help: eval('openHelp(222)')
      mask Display: image(imread('State.png'))
  STATE_BMW_Z3_Convertible_1_rc : RateTransition  Tag=mux_rc/StatePort  OutPortSampleTimeOpt=Inherit
  SteeringWheel_pivot_Mux : Subsystem  Tag=mux/Joint  mask(PreScan Mux Block){DisplayName=SteeringWheel}
      mask prompts: DisplayName "Display Name"
      mask help:
      | This block simulates a generic joint used for generic models. This joint can be enabled/disabled from the GUI.
      |
      | For more information, please click Help.
      settings: DeleteFcn=PreScanBlockDeleteFcn;
      mask Help: eval('openHelp(254)')
  Terminator_{1..13} (13 alike) : Terminator
  V2X_28_CAM_Expander : Subsystem  LoadFcn=addpath .\V2XPlugin; V2Xbusses;
  V2X_28_CAM_Filter : Subsystem
      mask Display: disp('[3]');
  V2X_Tx28_CAM : Subsystem
  V2X_Tx28_CAM_Enable : Constant  OutDataTypeStr=Inherit: Inherit via back propagation
  STATE_BMW_Z3_Convertible_1_bus : Outport  Tag=outport/StatePort  OutDataTypeStr=Bus: PRESCAN_STATEACTUATORDATA  PortDimensions=1  SampleTime=1/20
  SteeringWheel_pivot_BMW_Z3_Convertible_1 : Outport  Tag=outport/JointActuator  Port=2  OutDataTypeStr=Bus: PRESCAN_POSE_DATA  SampleTime=1/20
  V2X_Tx28_CAM_Transmitter : Outport  Tag=outport/plugin/sfun_V2X_CAM_Transmitter  Port=3
  wires:
  STATE_BMW_Z3_Convertible_1_rc/1 -> STATE_BMW_Z3_Convertible_1_bus/1
  STATE_BMW_Z3_Convertible_1/1(StateBus) -> STATE_BMW_Z3_Convertible_1_rc/1
  SELF_BMW_Z3_Convertible_1/1 -> SELF_Demux/1(SELF)
  SteeringWheel_pivot_Mux/1(Joint) -> SteeringWheel_pivot_BMW_Z3_Convertible_1/1
  Dynamics_Empty/1(State) -> STATE_BMW_Z3_Convertible_1/1(State)
  V2X_Tx28_CAM_Enable/1 -> V2X_Tx28_CAM/1(Enabled)
  V2X_Tx28_CAM/1(PRESCAN_V2X_USER_CAM_MESSAGE) -> V2X_28_CAM_Expander/1(In)
  V2X_28_CAM_Expander/1(Out) -> V2X_Tx28_CAM_Transmitter/1
  V2X_Rx28_CAM_Receiver/1 -> V2X_28_CAM_Filter/1(Filter_In)
  SELF_Demux/1(x [m]) -> Terminator_1/1
  SELF_Demux/2(y [m]) -> Terminator_2/1
  SELF_Demux/3(z [m]) -> Terminator_3/1
  SELF_Demux/4(rotx [deg]) -> Terminator_4/1
  SELF_Demux/5(roty [deg]) -> Terminator_5/1
  SELF_Demux/6(rotz [deg]) -> Terminator_6/1
  SELF_Demux/7(GPS lat [deg]) -> Terminator_7/1
  SELF_Demux/8(GPS long [deg]) -> Terminator_8/1
  SELF_Demux/9(GPS alt [m]) -> Terminator_9/1
  SELF_Demux/10(velocity [m/s]) -> Terminator_10/1
  SELF_Demux/11(heading [deg]) -> Terminator_11/1
  SELF_Demux/12(yaw rate [deg/s]) -> Terminator_12/1
  Ground_1/1 -> SteeringWheel_pivot_Mux/1(X [m])
  Ground_2/1 -> SteeringWheel_pivot_Mux/2(Y [m])
  Ground_3/1 -> SteeringWheel_pivot_Mux/3(Z [m])
  Ground_4/1 -> SteeringWheel_pivot_Mux/4(Roll [rad])
  Ground_5/1 -> SteeringWheel_pivot_Mux/5(Pitch [rad])
  Ground_6/1 -> SteeringWheel_pivot_Mux/6(Yaw [rad])
  V2X_28_CAM_Filter/1(Filter_Out) -> Terminator_13/1
  Ground_7/1 -> V2X_Tx28_CAM/2(DATA.h.protocolVersion)
  Ground_8/1 -> V2X_Tx28_CAM/3(DATA.h.messageID)
  Ground_9/1 -> V2X_Tx28_CAM/4(DATA.h.stationID)
  Ground_10/1 -> V2X_Tx28_CAM/5(DATA.c.generationDeltaTime)
  Ground_11/1 -> V2X_Tx28_CAM/6(DATA.c.cP.bC.stationType)
  Ground_12/1 -> V2X_Tx28_CAM/7(DATA.c.cP.bC.rP.latitude)
  Ground_13/1 -> V2X_Tx28_CAM/8(DATA.c.cP.bC.rP.longitude)
  Ground_14/1 -> V2X_Tx28_CAM/9(DATA.c.cP.bC.rP.pCE.semiMajorConfidence)
  Ground_15/1 -> V2X_Tx28_CAM/10(DATA.c.cP.bC.rP.pCE.semiMinorConfidence)
  Ground_16/1 -> V2X_Tx28_CAM/11(DATA.c.cP.bC.rP.pCE.semiMajorOrientation)
  Ground_17/1 -> V2X_Tx28_CAM/12(DATA.c.cP.bC.rP.a.altitudeValue)
  Ground_18/1 -> V2X_Tx28_CAM/13(DATA.c.cP.bC.rP.a.altitudeConfidence)
  Ground_19/1 -> V2X_Tx28_CAM/14(DATA.c.cP.hFC.bVCHF.h.headingValue)
  Ground_20/1 -> V2X_Tx28_CAM/15(DATA.c.cP.hFC.bVCHF.h.headingConfidence)
  Ground_21/1 -> V2X_Tx28_CAM/16(DATA.c.cP.hFC.bVCHF.s.speedValue)
  Ground_22/1 -> V2X_Tx28_CAM/17(DATA.c.cP.hFC.bVCHF.s.speedConfidence)
  Ground_23/1 -> V2X_Tx28_CAM/18(DATA.c.cP.hFC.bVCHF.driveDirection)
  Ground_24/1 -> V2X_Tx28_CAM/19(DATA.c.cP.hFC.bVCHF.vL.vehicleLengthValue)
  Ground_25/1 -> V2X_Tx28_CAM/20(DATA.c.cP.hFC.bVCHF.vL.vehicleLengthConfidenceIndication)
  Ground_26/1 -> V2X_Tx28_CAM/21(DATA.c.cP.hFC.bVCHF.vehicleWidth)
  Ground_27/1 -> V2X_Tx28_CAM/22(DATA.c.cP.hFC.bVCHF.lA.longitudinalAccelerationValue)
  Ground_28/1 -> V2X_Tx28_CAM/23(DATA.c.cP.hFC.bVCHF.lA.longitudinalAccelerationConfidence)
  Ground_29/1 -> V2X_Tx28_CAM/24(DATA.c.cP.hFC.bVCHF.c.curvatureValue)
  Ground_30/1 -> V2X_Tx28_CAM/25(DATA.c.cP.hFC.bVCHF.c.curvatureConfidence)
  Ground_31/1 -> V2X_Tx28_CAM/26(DATA.c.cP.hFC.bVCHF.curvatureCalculationMode)
  Ground_32/1 -> V2X_Tx28_CAM/27(DATA.c.cP.hFC.bVCHF.yR.yawRateValue)
  Ground_33/1 -> V2X_Tx28_CAM/28(DATA.c.cP.hFC.bVCHF.yR.yawRateConfidence)

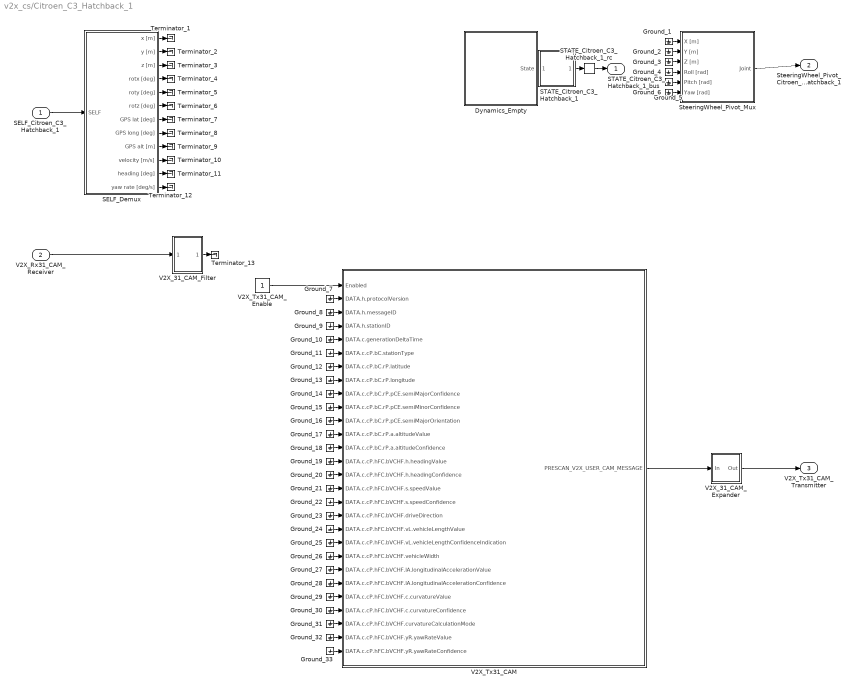
== system v2x_cs/Citroen_C3_Hatchback_1 ==
  SELF_Citroen_C3_Hatchback_1 : Inport  Tag=inport/SelfPort  OutDataTypeStr=Bus: PRESCAN_SELFSENSORDATA  PortDimensions=1  SampleTime=1/20  BusOutputAsStruct=on
  V2X_Rx31_CAM_Receiver : Inport  Tag=inport/plugin/sfun_V2X_CAM_Receiver  Port=2  BusOutputAsStruct=on
  Dynamics_Empty : Subsystem  Tag=Dynamics_Empty
      mask Help: eval('openHelp(202)')
      mask Display: port_label('output', 1, 'State');text(0,0,' Empty\n')
  Ground_{1..33} (33 alike) : Ground
  SELF_Demux : Subsystem  Tag=demux/SelfPort  mask(PreScan Demux Block:){}
      mask help:
      | The SELF port shows (state) information of the actor itself. The outputs are position in the experiment's axis system and the GPS coordinates, and the object's absolute velocity and compass heading.
      |
      | For more information, please click Help.
      settings: DeleteFcn=PreScanBlockDeleteFcn;
      mask Help: eval('openHelp(462)')
      mask Display:
      | port_label('output',1,'x [m]')
      | port_label('output',2,'y [m]')
      | port_label('output',3,'z [m]','texmode','on')
      | port_label('output',4,'Rotx [deg]','texmode','on')
      | port_label('output',5,'Roty [deg]','texmode','on')
      | port_label('output',6,'Rotz [deg]','texmode','on')
      | port_label('output',7,'GPS lat [deg]','texmode','on')
      | port_label('output',8,'GPS long [deg]','texmode','on')
      | port_label('output',9,'GPS alt [m]','texmode','on')
      | port_label('output',10,'Velocity [m/s]')
      | port_label('output',11,'Heading [deg]')
      | port_label('output',12,'Yaw rate [deg/s]')
  STATE_Citroen_C3_Hatchback_1 : Subsystem  Tag=mux/StatePort  Priority=0  LoadFcn=load PrescanStateActuatorData  mask(PreScan Sink Block: State){x0=30.9394, y0=-4.3798, z0=0.58, Roll0=0, Pitch0=0, Yaw0=0, TimeStep=1/20}
      mask prompts: x0 "Ini x-position VEHICLE wrt GLOBAL axis system [m]"; y0 "Ini y-position VEHICLE wrt GLOBAL axis system [m]"; z0 "Ini z-position VEHICLE wrt GLOBAL axis system [m]"; Roll0 "Ini roll-angle BODY wrt VEHICLE axis system [deg]"; Pitch0 "Ini pitch-angle BODY wrt VEHICLE axis system [deg]"; Yaw0 "Ini yaw-angle VEHICLE wrt GLOBAL axis system [deg]"; TimeStep "Auto-Assigned: Upload Period [s]"
      mask help:
      | The Actor State contains a vector signal of size (9x1), containing the following signals:
      |
      | -  Position                  (x,y,z)                                     [m]
      | -  Velocity                  (vx,vy,vz)                               [m/s]
      | -  Angles                    (Roll, Pitch, Yaw)                   [rad]
      |
      | The Actor state is defined in the global axis system.
      | The state is superponed on the Initial position defined in the GUI.
      |
      | For more information, please click Help.
      settings: DeleteFcn=PreScanBlockDeleteFcn;
      mask Help: eval('openHelp(222)')
      mask Display: image(imread('State.png'))
  STATE_Citroen_C3_Hatchback_1_rc : RateTransition  Tag=mux_rc/StatePort  OutPortSampleTimeOpt=Inherit
  SteeringWheel_Pivot_Mux : Subsystem  Tag=mux/Joint  mask(PreScan Mux Block){DisplayName=SteeringWheel}
      mask prompts: DisplayName "Display Name"
      mask help:
      | This block simulates a generic joint used for generic models. This joint can be enabled/disabled from the GUI.
      |
      | For more information, please click Help.
      settings: DeleteFcn=PreScanBlockDeleteFcn;
      mask Help: eval('openHelp(254)')
  Terminator_{1..13} (13 alike) : Terminator
  V2X_31_CAM_Expander : Subsystem  LoadFcn=addpath .\V2XPlugin; V2Xbusses;
  V2X_31_CAM_Filter : Subsystem
      mask Display: disp('[3]');
  V2X_Tx31_CAM : Subsystem
  V2X_Tx31_CAM_Enable : Constant  OutDataTypeStr=Inherit: Inherit via back propagation
  STATE_Citroen_C3_Hatchback_1_bus : Outport  Tag=outport/StatePort  OutDataTypeStr=Bus: PRESCAN_STATEACTUATORDATA  PortDimensions=1  SampleTime=1/20
  SteeringWheel_Pivot_Citroen_C3_Hatchback_1 : Outport  Tag=outport/JointActuator  Port=2  OutDataTypeStr=Bus: PRESCAN_POSE_DATA  SampleTime=1/20
  V2X_Tx31_CAM_Transmitter : Outport  Tag=outport/plugin/sfun_V2X_CAM_Transmitter  Port=3
  wires:
  STATE_Citroen_C3_Hatchback_1_rc/1 -> STATE_Citroen_C3_Hatchback_1_bus/1
  STATE_Citroen_C3_Hatchback_1/1(StateBus) -> STATE_Citroen_C3_Hatchback_1_rc/1
  SELF_Citroen_C3_Hatchback_1/1 -> SELF_Demux/1(SELF)
  SteeringWheel_Pivot_Mux/1(Joint) -> SteeringWheel_Pivot_Citroen_C3_Hatchback_1/1
  Dynamics_Empty/1(State) -> STATE_Citroen_C3_Hatchback_1/1(State)
  V2X_Tx31_CAM_Enable/1 -> V2X_Tx31_CAM/1(Enabled)
  V2X_Tx31_CAM/1(PRESCAN_V2X_USER_CAM_MESSAGE) -> V2X_31_CAM_Expander/1(In)
  V2X_31_CAM_Expander/1(Out) -> V2X_Tx31_CAM_Transmitter/1
  V2X_Rx31_CAM_Receiver/1 -> V2X_31_CAM_Filter/1(Filter_In)
  SELF_Demux/1(x [m]) -> Terminator_1/1
  SELF_Demux/2(y [m]) -> Terminator_2/1
  SELF_Demux/3(z [m]) -> Terminator_3/1
  SELF_Demux/4(rotx [deg]) -> Terminator_4/1
  SELF_Demux/5(roty [deg]) -> Terminator_5/1
  SELF_Demux/6(rotz [deg]) -> Terminator_6/1
  SELF_Demux/7(GPS lat [deg]) -> Terminator_7/1
  SELF_Demux/8(GPS long [deg]) -> Terminator_8/1
  SELF_Demux/9(GPS alt [m]) -> Terminator_9/1
  SELF_Demux/10(velocity [m/s]) -> Terminator_10/1
  SELF_Demux/11(heading [deg]) -> Terminator_11/1
  SELF_Demux/12(yaw rate [deg/s]) -> Terminator_12/1
  Ground_1/1 -> SteeringWheel_Pivot_Mux/1(X [m])
  Ground_2/1 -> SteeringWheel_Pivot_Mux/2(Y [m])
  Ground_3/1 -> SteeringWheel_Pivot_Mux/3(Z [m])
  Ground_4/1 -> SteeringWheel_Pivot_Mux/4(Roll [rad])
  Ground_5/1 -> SteeringWheel_Pivot_Mux/5(Pitch [rad])
  Ground_6/1 -> SteeringWheel_Pivot_Mux/6(Yaw [rad])
  V2X_31_CAM_Filter/1(Filter_Out) -> Terminator_13/1
  Ground_7/1 -> V2X_Tx31_CAM/2(DATA.h.protocolVersion)
  Ground_8/1 -> V2X_Tx31_CAM/3(DATA.h.messageID)
  Ground_9/1 -> V2X_Tx31_CAM/4(DATA.h.stationID)
  Ground_10/1 -> V2X_Tx31_CAM/5(DATA.c.generationDeltaTime)
  Ground_11/1 -> V2X_Tx31_CAM/6(DATA.c.cP.bC.stationType)
  Ground_12/1 -> V2X_Tx31_CAM/7(DATA.c.cP.bC.rP.latitude)
  Ground_13/1 -> V2X_Tx31_CAM/8(DATA.c.cP.bC.rP.longitude)
  Ground_14/1 -> V2X_Tx31_CAM/9(DATA.c.cP.bC.rP.pCE.semiMajorConfidence)
  Ground_15/1 -> V2X_Tx31_CAM/10(DATA.c.cP.bC.rP.pCE.semiMinorConfidence)
  Ground_16/1 -> V2X_Tx31_CAM/11(DATA.c.cP.bC.rP.pCE.semiMajorOrientation)
  Ground_17/1 -> V2X_Tx31_CAM/12(DATA.c.cP.bC.rP.a.altitudeValue)
  Ground_18/1 -> V2X_Tx31_CAM/13(DATA.c.cP.bC.rP.a.altitudeConfidence)
  Ground_19/1 -> V2X_Tx31_CAM/14(DATA.c.cP.hFC.bVCHF.h.headingValue)
  Ground_20/1 -> V2X_Tx31_CAM/15(DATA.c.cP.hFC.bVCHF.h.headingConfidence)
  Ground_21/1 -> V2X_Tx31_CAM/16(DATA.c.cP.hFC.bVCHF.s.speedValue)
  Ground_22/1 -> V2X_Tx31_CAM/17(DATA.c.cP.hFC.bVCHF.s.speedConfidence)
  Ground_23/1 -> V2X_Tx31_CAM/18(DATA.c.cP.hFC.bVCHF.driveDirection)
  Ground_24/1 -> V2X_Tx31_CAM/19(DATA.c.cP.hFC.bVCHF.vL.vehicleLengthValue)
  Ground_25/1 -> V2X_Tx31_CAM/20(DATA.c.cP.hFC.bVCHF.vL.vehicleLengthConfidenceIndication)
  Ground_26/1 -> V2X_Tx31_CAM/21(DATA.c.cP.hFC.bVCHF.vehicleWidth)
  Ground_27/1 -> V2X_Tx31_CAM/22(DATA.c.cP.hFC.bVCHF.lA.longitudinalAccelerationValue)
  Ground_28/1 -> V2X_Tx31_CAM/23(DATA.c.cP.hFC.bVCHF.lA.longitudinalAccelerationConfidence)
  Ground_29/1 -> V2X_Tx31_CAM/24(DATA.c.cP.hFC.bVCHF.c.curvatureValue)
  Ground_30/1 -> V2X_Tx31_CAM/25(DATA.c.cP.hFC.bVCHF.c.curvatureConfidence)
  Ground_31/1 -> V2X_Tx31_CAM/26(DATA.c.cP.hFC.bVCHF.curvatureCalculationMode)
  Ground_32/1 -> V2X_Tx31_CAM/27(DATA.c.cP.hFC.bVCHF.yR.yawRateValue)
  Ground_33/1 -> V2X_Tx31_CAM/28(DATA.c.cP.hFC.bVCHF.yR.yawRateConfidence)
